simulink model "Convert_RPM_Radian"  (R2021a)
settings: Solver=VariableStepAuto  StartTime=0.0  StopTime=10.0  RelTol=1e-3
settings Model: Creator=my computer  LastModifiedBy=my computer

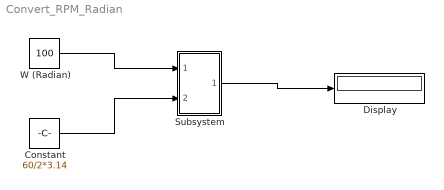
== system Convert_RPM_Radian ==
  Constant : Constant  Value=60/2*3.14
  Display : Display
  Subsystem : Subsystem
  W (Radian) : Constant  Value=100
  wires:
  W (Radian)/1 -> Subsystem/1(In1)
  Constant/1 -> Subsystem/2(In2)
  Subsystem/1(Out1) -> Display/1

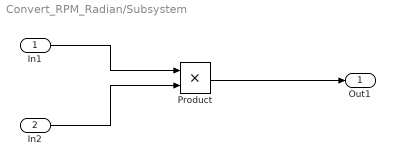
== system Convert_RPM_Radian/Subsystem ==
  In1 : Inport
  In2 : Inport  Port=2
  Product : Product
  Out1 : Outport
  wires:
  Product/1 -> Out1/1
  In1/1 -> Product/1
  In2/1 -> Product/2
